simulink model "Lab1_simscape"  (R2021a)
settings: Solver=VariableStepAuto  StartTime=0.0  StopTime=t  MaxStep=1e-3  RelTol=1e-3
undefined symbols (not defined in the file): A_1, A_2, b1, b2, b3, T_1, T_2, x1_0, x2_0
libraries: fl_lib x20, nesl_utility x13
settings Model: Creator=User  LastModifiedBy=Alex

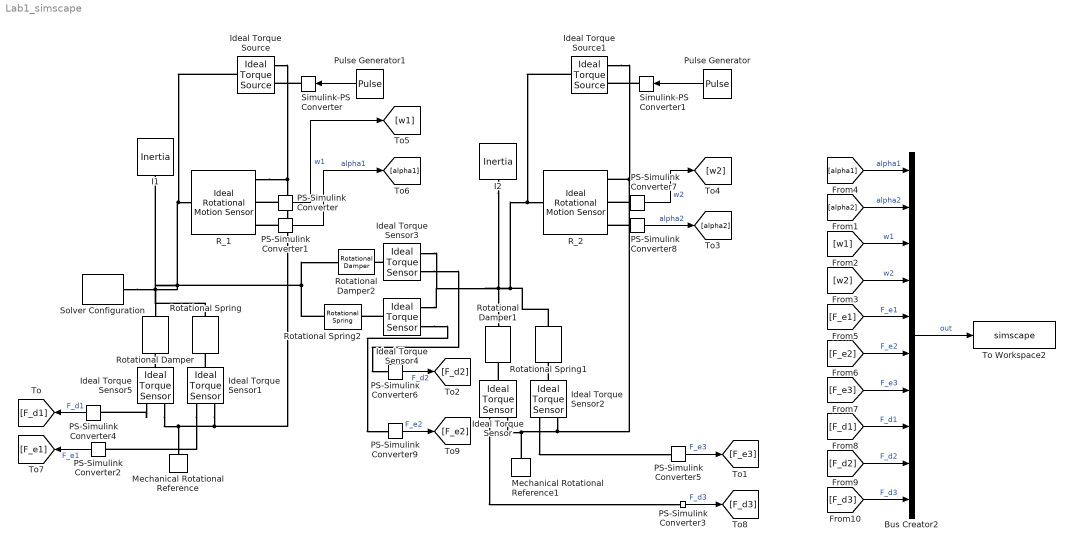
== system Lab1_simscape ==
  Bus Creator2 : BusCreator  Inputs=10
  I1 : fl_lib/Mechanical/Rotational Elements/Inertia  inertia=I1 kg*m^2  num_ports=foundation.enum.numPorts2.one  w_specify=off  w_priority=High  w=0 rad/s  w_nominal_specify=off  w_nominal_unit=rad/s  w_nominal_value=1  t_specify=off  t_priority=None  t=0 N*m  t_nominal_specify=off  t_nominal_unit=N*m  t_nominal_value=1
  I2 : fl_lib/Mechanical/Rotational Elements/Inertia  inertia=I1 kg*m^2  num_ports=foundation.enum.numPorts2.one  w_specify=off  w_priority=High  w=0 rad/s  w_nominal_specify=off  w_nominal_unit=rad/s  w_nominal_value=1  t_specify=off  t_priority=None  t=0 N*m  t_nominal_specify=off  t_nominal_unit=N*m  t_nominal_value=1
  Ideal Torque Sensor{,1..5} (6 alike) : fl_lib/Mechanical/Mechanical Sensors/Ideal Torque Sensor
  Ideal Torque Source : fl_lib/Mechanical/Mechanical Sources/Ideal Torque Source
  Ideal Torque Source1 : fl_lib/Mechanical/Mechanical Sources/Ideal Torque Source
  Mechanical Rotational Reference : fl_lib/Mechanical/Rotational Elements/Mechanical Rotational Reference
  Mechanical Rotational Reference1 : fl_lib/Mechanical/Rotational Elements/Mechanical Rotational Reference
  PS-Simulink Converter{,1..9} (10 alike) : nesl_utility/PS-Simulink Converter  PhysicalDomain=network_engine_domain  SubClassName=ps_output  LeftPortType=input  RightPortType=output  PseudoPeriodic=off  Frequencies=[]  Unit=inherit  AffineConversion=off
      settings: SourceProductBaseCode=PW,SS
  Pulse Generator : DiscretePulseGenerator  PulseType=Time based  Amplitude=A_2  Period=T_2  PulseWidth=(0.5/T_2) * 100
  Pulse Generator1 : DiscretePulseGenerator  PulseType=Time based  Amplitude=A_1  Period=T_1  PulseWidth=(0.5/T_1) * 100
  R_1 : fl_lib/Mechanical/Mechanical Sensors/Ideal Rotational Motion Sensor  wrap_angle=simscape.enum.onoff.off  offset=x1_0 rad
  R_2 : fl_lib/Mechanical/Mechanical Sensors/Ideal Rotational Motion Sensor  wrap_angle=simscape.enum.onoff.off  offset=x2_0 rad
  Rotational Damper : fl_lib/Mechanical/Rotational Elements/Rotational Damper  D=b1 N*m/(rad/s)  w_specify=off  w_priority=None  w=0 rad/s  w_nominal_specify=off  w_nominal_unit=rad/s  w_nominal_value=1  t_specify=off  t_priority=None  t=0 N*m  t_nominal_specify=off  t_nominal_unit=N*m  t_nominal_value=1
  Rotational Damper1 : fl_lib/Mechanical/Rotational Elements/Rotational Damper  D=b3 N*m/(rad/s)  w_specify=off  w_priority=None  w=0 rad/s  w_nominal_specify=off  w_nominal_unit=rad/s  w_nominal_value=1  t_specify=off  t_priority=None  t=0 N*m  t_nominal_specify=off  t_nominal_unit=N*m  t_nominal_value=1
  Rotational Damper2 : fl_lib/Mechanical/Rotational Elements/Rotational Damper  D=b2 N*m/(rad/s)  w_specify=off  w_priority=None  w=0 rad/s  w_nominal_specify=off  w_nominal_unit=rad/s  w_nominal_value=1  t_specify=off  t_priority=None  t=0 N*m  t_nominal_specify=off  t_nominal_unit=N*m  t_nominal_value=1
  Rotational Spring : fl_lib/Mechanical/Rotational Elements/Rotational Spring  spr_rate=k1 N*m/rad  w_specify=off  w_priority=None  w=0 rad/s  w_nominal_specify=off  w_nominal_unit=rad/s  w_nominal_value=1  t_specify=off  t_priority=None  t=0 N*m  t_nominal_specify=off  t_nominal_unit=N*m  t_nominal_value=1  phi_specify=on  phi_priority=High  phi=x1_0 rad  phi_nominal_specify=off  phi_nominal_unit=rad  phi_nominal_value=1
  Rotational Spring1 : fl_lib/Mechanical/Rotational Elements/Rotational Spring  spr_rate=k3 N*m/rad  w_specify=off  w_priority=None  w=0 rad/s  w_nominal_specify=off  w_nominal_unit=rad/s  w_nominal_value=1  t_specify=off  t_priority=None  t=0 N*m  t_nominal_specify=off  t_nominal_unit=N*m  t_nominal_value=1  phi_specify=on  phi_priority=High  phi=x2_0 rad  phi_nominal_specify=off  phi_nominal_unit=rad  phi_nominal_value=1
  Rotational Spring2 : fl_lib/Mechanical/Rotational Elements/Rotational Spring  spr_rate=k2 N*m/rad  w_specify=off  w_priority=None  w=0 rad/s  w_nominal_specify=off  w_nominal_unit=rad/s  w_nominal_value=1  t_specify=off  t_priority=None  t=0 N*m  t_nominal_specify=off  t_nominal_unit=N*m  t_nominal_value=1  phi_specify=on  phi_priority=High  phi=x2_0-x1_0 rad  phi_nominal_specify=off  phi_nominal_unit=rad  phi_nominal_value=1
  Simulink-PS Converter : nesl_utility/Simulink-PS Converter  PhysicalDomain=network_engine_domain  SubClassName=ps_input  LeftPortType=input  RightPortType=output  PseudoPeriodic=off  Frequencies=[]  NoiseDistribution=none  NoiseParameters=[]  Unit=1  AffineConversion=off  FilteringAndDerivatives=provide  SimscapeFilterOrder=1  InputFilterTimeConstant=0.001  UdotUserProvided=0
      settings: SourceProductBaseCode=PW,SS
  Simulink-PS Converter1 : nesl_utility/Simulink-PS Converter  PhysicalDomain=network_engine_domain  SubClassName=ps_input  LeftPortType=input  RightPortType=output  PseudoPeriodic=off  Frequencies=[]  NoiseDistribution=none  NoiseParameters=[]  Unit=1  AffineConversion=off  FilteringAndDerivatives=provide  SimscapeFilterOrder=1  InputFilterTimeConstant=0.001  UdotUserProvided=0
      settings: SourceProductBaseCode=PW,SS
  Solver Configuration : nesl_utility/Solver Configuration  PhysicalDomain=network_engine_domain  SubClassName=solver  LeftPortType=input  RightPortType=generic  Tones=[]  Harmonics=[]  SimulateNoise=off  Profile=off  UseLocalSampling=off  EnableSwitchedLinearOptims=on  FrequencyDomain=off  UseCCode=off  RelTol=0.001  AbsTol=1e-06  MinStep=1e-09  ToWorkspace=off  RevertToSquareIcSolve=off  NumHomotopyIterations=100  PhasorMode=off  PhasorModeNumHarmonics=1  DoDC=off  ResidualTolerance=1e-09  UseLocalSolver=off  LocalSolverChoice=NE_BACKWARD_EULER_ADVANCER  LocalSolverSampleTime=0.001  DoFixedCost=off  MaxNonlinIter=3  MaxModeIter=2  ComputeImpulses=off  ImpulseIterations=2  LinearAlgebra=auto  EquationFormulation=NE_TIME_EF  DelaysMemoryBudget=1024  AutomaticFiltering=on  FilteringTimeConstant=0.001  PartitionStorageMethod=AS_NEEDED  PartitionMemoryBudget=1024  PartitionMethod=ROBUST
      settings: SourceProductBaseCode=PW,SS
  To Workspace2 : ToWorkspace  VariableName=simscape  SaveFormat=Timeseries  SampleTime=-1
  wires:
  PS-Simulink Converter4/1 -> [F_d1]  "F_d1"
  PS-Simulink Converter5/1 -> [F_e3]  "F_e3"
  PS-Simulink Converter6/1 -> [F_d2]  "F_d2"
  PS-Simulink Converter8/1 -> [alpha2]  "alpha2"
  PS-Simulink Converter7/1 -> [w2]  "w2"
  PS-Simulink Converter/1 -> [w1]  "w1"
  PS-Simulink Converter1/1 -> [alpha1]  "alpha1"
  Bus Creator2/1 -> To Workspace2/1  "out"
  [alpha1] -> Bus Creator2/1  "alpha1"
  [alpha2] -> Bus Creator2/2  "alpha2"
  [w1] -> Bus Creator2/3  "w1"
  [w2] -> Bus Creator2/4  "w2"
  [F_e1] -> Bus Creator2/5  "F_e1"
  [F_e2] -> Bus Creator2/6  "F_e2"
  [F_e3] -> Bus Creator2/7  "F_e3"
  PS-Simulink Converter2/1 -> [F_e1]  "F_e1"
  PS-Simulink Converter3/1 -> [F_d3]  "F_d3"
  PS-Simulink Converter9/1 -> [F_e2]  "F_e2"
  [F_d1] -> Bus Creator2/8  "F_d1"
  [F_d2] -> Bus Creator2/9  "F_d2"
  [F_d3] -> Bus Creator2/10  "F_d3"
  Pulse Generator/1 -> Simulink-PS Converter1/1
  Pulse Generator1/1 -> Simulink-PS Converter/1
  connections:
  Rotational Spring2/RConn1 -- Rotational Damper2/RConn1 -- Ideal Torque Source/LConn1 -- R_1/LConn1 -- Rotational Spring/LConn1 -- Rotational Damper/LConn1 -- Solver Configuration/RConn1 -- I1/LConn1
  Mechanical Rotational Reference1/LConn1 -- Ideal Torque Sensor/RConn1 -- Ideal Torque Sensor2/RConn1 -- Ideal Torque Source1/RConn2 -- R_2/RConn1
  Rotational Spring1/LConn1 -- Rotational Damper1/LConn1 -- Ideal Torque Sensor3/RConn1 -- Ideal Torque Sensor4/RConn1 -- I2/LConn1 -- Ideal Torque Source1/LConn1 -- R_2/LConn1
  R_1/RConn1 -- Ideal Torque Source/RConn2 -- Ideal Torque Sensor1/RConn1 -- Ideal Torque Sensor5/RConn1 -- Mechanical Rotational Reference/LConn1
  PS-Simulink Converter/LConn1 -- R_1/RConn2
  PS-Simulink Converter1/LConn1 -- R_1/RConn3
  PS-Simulink Converter7/LConn1 -- R_2/RConn2
  PS-Simulink Converter8/LConn1 -- R_2/RConn3
  Ideal Torque Sensor3/LConn1 -- Rotational Damper2/LConn1
  Ideal Torque Sensor4/LConn1 -- Rotational Spring2/LConn1
  Ideal Torque Sensor3/RConn2 -- PS-Simulink Converter6/LConn1
  Ideal Torque Sensor4/RConn2 -- PS-Simulink Converter9/LConn1
  Ideal Torque Sensor5/LConn1 -- Rotational Damper/RConn1
  Ideal Torque Sensor1/LConn1 -- Rotational Spring/RConn1
  Ideal Torque Sensor5/RConn2 -- PS-Simulink Converter4/LConn1
  Ideal Torque Sensor1/RConn2 -- PS-Simulink Converter2/LConn1
  Ideal Torque Sensor/LConn1 -- Rotational Damper1/RConn1
  Ideal Torque Sensor2/LConn1 -- Rotational Spring1/RConn1
  Ideal Torque Sensor2/RConn2 -- PS-Simulink Converter5/LConn1
  Ideal Torque Sensor/RConn2 -- PS-Simulink Converter3/LConn1
  Simulink-PS Converter/RConn1 -- Ideal Torque Source/RConn1
  Simulink-PS Converter1/RConn1 -- Ideal Torque Source1/RConn1
